simulink model "DeadbeatDisturbed"  (R2023a)
settings: Solver=VariableStepAuto  StartTime=0.0  StopTime=10.0  RelTol=1e-3
libraries: simulink x2
settings Model: Creator=bl4ck  LastModifiedBy=bl4ck

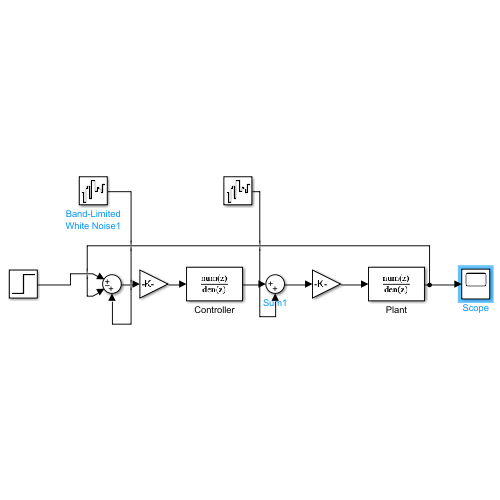
[thumbnail: Simulink's stored preview of the top-level diagram]
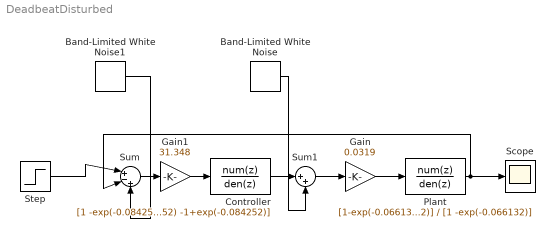
== system DeadbeatDisturbed ==
  Band-Limited White Noise : simulink/Sources/Band-Limited White Noise  Cov=[0.01]  Ts=0.01  seed=[23341]
  Band-Limited White Noise1 : simulink/Sources/Band-Limited White Noise  Cov=[0.01]  Ts=0.01  seed=[23341]
  Controller : DiscreteTransferFcn  Numerator=[1 -exp(-0.084252)]  Denominator=[1-exp(-0.084252) -1+exp(-0.084252)]  SampleTime=0.01274
  Gain : Gain  Gain=0.0319
  Gain1 : Gain  Gain=31.348
  Plant : DiscreteTransferFcn  Numerator=[1-exp(-0.066132)]  Denominator=[1 -exp(-0.066132)]  SampleTime=0.01274
  Scope : Scope
  Step : Step  After=10  SampleTime=0
  Sum : Sum  Inputs=|+-+
  Sum1 : Sum  Inputs=|++
  wires:
  Step/1 -> Sum/1
  Gain/1 -> Plant/1
  Plant/1 -> Sum/2, Scope/1
  Sum/1 -> Gain1/1
  Gain1/1 -> Controller/1
  Controller/1 -> Sum1/1
  Sum1/1 -> Gain/1
  Band-Limited White Noise1/1 -> Sum/3
  Band-Limited White Noise/1 -> Sum1/2
